simulink model "PV_Array_FLC"  (R2021a)
settings: Solver=VariableStepAuto  StartTime=0.0  StopTime=10.0  RelTol=1e-3
libraries: spsSeriesRLCBranchLib x3, spsDiodeLib x2, fuzblock x1, spsPWMGeneratorDCDCLib x1, spsMosfetLib x1, spsPVArrayLib x1, spsSeriesRLCLoadLib x1, spsVoltageMeasurementLib x1, spspowerguiLib x1
settings Model: Creator=admin  LastModifiedBy=admin

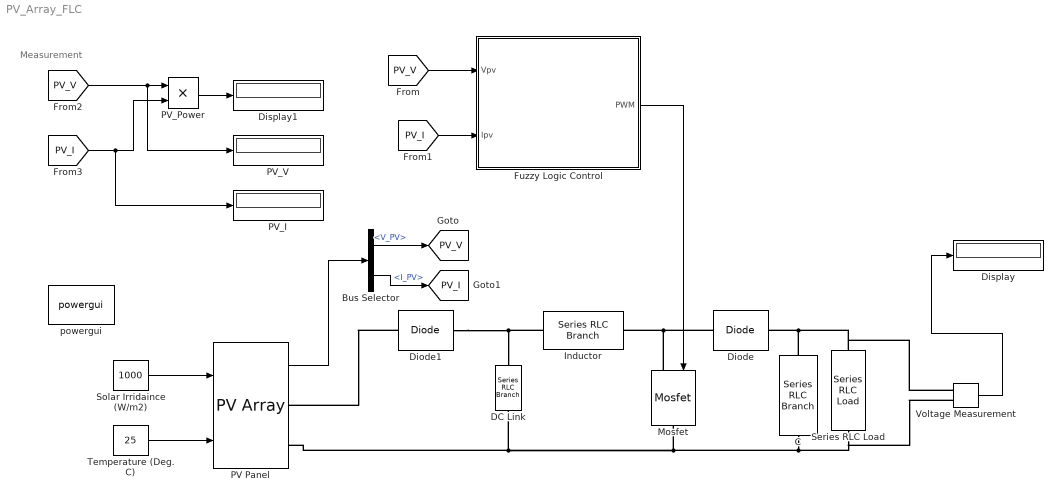
== system PV_Array_FLC ==
  note: Measurement
  Bus Selector : BusSelector  OutputSignals=V_PV,I_PV
  C : spsSeriesRLCBranchLib/Series RLC Branch  LConnTagsString=__new0  RConnTagsString=__new0  BranchType=C  Resistance=1  Inductance=1e-3  SetiL0=off  InitialCurrent=0  Capacitance=50e-6  Setx0=off  InitialVoltage=600  Measurements=None
  DC Link : spsSeriesRLCBranchLib/Series RLC Branch  LConnTagsString=__new0  RConnTagsString=__new0  BranchType=C  Resistance=0.001  Inductance=1.0  SetiL0=off  InitialCurrent=0  Capacitance=4000e-6  Setx0=off  InitialVoltage=310  Measurements=None
  Diode : spsDiodeLib/Diode  Ron=0.001  Lon=0  Vf=0.8  IC=0  UseSnubber=off  Rs=500  Cs=250e-9  Measurements=off
  Diode1 : spsDiodeLib/Diode  Ron=0.001  Lon=0  Vf=0.8  IC=0  UseSnubber=off  Rs=500  Cs=250e-9  Measurements=off
  Display : Display
  Display1 : Display
  "Fuzzy Logic Control " : Subsystem
  Inductor : spsSeriesRLCBranchLib/Series RLC Branch  LConnTagsString=__new0  RConnTagsString=__new0  BranchType=L  Resistance=0.01  Inductance=4e-4  SetiL0=off  InitialCurrent=5  Capacitance=1e-6  Setx0=off  InitialVoltage=0  Measurements=None
  Mosfet : spsMosfetLib/Mosfet  Ron=0.1  Lon=0  Rd=0.01  Vfd=0  IC=0  Rs=1e5  Cs=inf  Measurements=off
  "PV Panel  " : spsPVArrayLib/PV Array  Npar=1  Nser=2  PlotType=array @ 25 deg.C & specified irradiances  S_vec="[ 1000  500  100 ]"  Temp_C_vec="[ 45 25  ]"  ModuleName=Aavid Solar ASMS-220P  PlotWhenSelected=off  Pm=220.5  Ncell=60  Voc=36.8  Isc=8.08  Vm=30  Im=7.35  beta_Voc_pc=-0.3364  alpha_Isc_pc=0.038465  beta_Voc=-0.1238  alpha_Isc=0.003108  IL=8.1108  I0=1.1169e-10  nI=0.9567  Rsh=83.699  Rs=0.3192  RobustModel=off  RobustCellTemperature=313.3991  BAL=on  Tc=1e-6  Tfilter=5e-5
  PV_I : Display
  "PV_Power " : Product
  PV_V : Display
  Series RLC Load : spsSeriesRLCLoadLib/Series RLC Load  LConnTagsString=a  RConnTagsString=__new0  NominalVoltage=30  NominalFrequency=50  ActivePower=120  InductivePower=0  CapacitivePower=0  Setx0=off  InitialVoltage=0  SetiL0=off  InitialCurrent=0  Measurements=None  LoadType=constant Z
  Solar Irridaince (W/m2) : Constant  Value=1000
  Temperature (Deg. C) : Constant  Value=25
  Voltage Measurement : spsVoltageMeasurementLib/Voltage Measurement  PhasorSimulation=off  OutputType=Complex  PSBequivalent=0
  powergui : spspowerguiLib/powergui  Priority=1  SimulationMode=Discrete  SampleTime=5e-7  frequency=60  Iterations=50  frequencyindice=0  Pbase=100e6  ErrMax=1e-4  UnitsV=kV  UnitsW=MW  buscounter=0  FunctionMessages=off  echomessages=off  EnableUseOfTLC=off  CurrentSourceSwitches=off  DisableSnubberDevices=off  DisableRonSwitches=off  DisableVfSwitches=off  DisplayEquations=off  AutomaticDiscreteSolvers=off  SolverType=Tustin/Backward Euler (TBE)  Interpol=off  ExternalGateDelay=off  methode=off  Ts=100  x0status=blocks  SPID=off  SwTol=0  HookPort=off  NonlinearTolerance=1e-4  nMaxIteration=100  ContinueOnMaxIteration=off  RestoreLinks=warning  ResistiveCurrentMeasurement=off  Frange=[0:2:500]  Ylog=off  Xlog=on  ShowGrid=off  save=off  variable=ZData  structure=0  ZoomFFT=off  StartTime=0.0  cycles=1  DisplayStyle=1  fundamental=60  FreqAxis=off  MaxFrequency=1000  frequencyindicesteady=1  RmsSteady=1  display=off
  tag scope: PV_I=global, PV_V=global
  wires:
  "Fuzzy Logic Control "/1(PWM) -> Mosfet/1
  Temperature (Deg. C)/1 -> "PV Panel  "/2
  Solar Irridaince (W/m2)/1 -> "PV Panel  "/1
  Bus Selector/1 -> [PV_V]  "<V_PV>"
  Bus Selector/2 -> [PV_I]  "<I_PV>"
  [PV_V] -> "Fuzzy Logic Control "/1(Vpv)
  [PV_I] -> "Fuzzy Logic Control "/2(Ipv)
  "PV Panel  "/1 -> Bus Selector/1
  [PV_V] -> PV_V/1, "PV_Power "/1
  [PV_I] -> PV_I/1, "PV_Power "/2
  "PV_Power "/1 -> Display1/1
  Voltage Measurement/1 -> Display/1
  connections:
  Mosfet/RConn1 -- Voltage Measurement/LConn2 -- Series RLC Load/RConn1 -- C/RConn1 -- DC Link/RConn1 -- "PV Panel  "/RConn2
  C/LConn1 -- Voltage Measurement/LConn1 -- Series RLC Load/LConn1 -- Diode/RConn1
  Diode1/RConn1 -- DC Link/LConn1 -- Inductor/LConn1
  Mosfet/LConn1 -- Inductor/RConn1 -- Diode/LConn1
  Diode1/LConn1 -- "PV Panel  "/RConn1

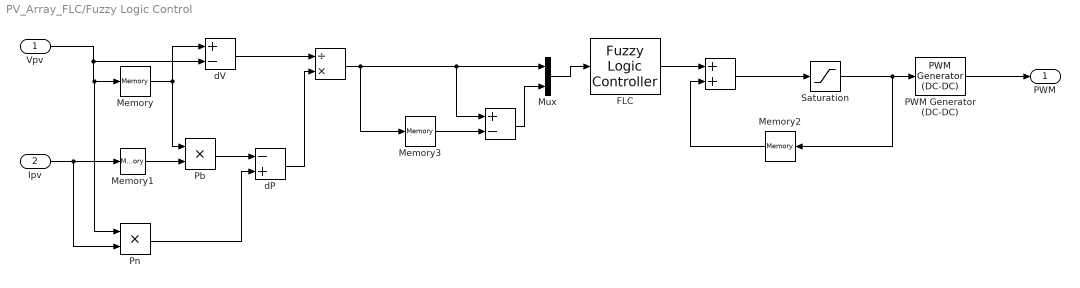
== system PV_Array_FLC/Fuzzy Logic Control  ==
  Vpv : Inport
  Ipv : Inport  Port=2
  "  " : Sum  Inputs=+-
  "   " : Sum
  "    " : Product  Inputs=/*
  "FLC " : fuzblock/Fuzzy Logic  Controller  FIS='tipper.fis'  OutputSampleNumber=101  DataType=double  FuzzifiedInputs=off  RuleFiringStrengths=off  RuleOutputs=off  AggregatedOutputs=off  SimulateUsing=Interpreted execution  OutOfRangeInputValueMessage=warning  NoRuleFiredMessage=warning  EmptyOutputFuzzySetMessage=warning
  "Memory " : Memory  InheritSampleTime=on
  "Memory1 " : Memory  InheritSampleTime=on
  Memory2 : Memory  InheritSampleTime=on
  Memory3 : Memory  InheritSampleTime=on
  Mux : Mux  Inputs=2
  PWM Generator (DC-DC) : spsPWMGeneratorDCDCLib/PWM Generator (DC-DC)  Fsw=15000  Ts=0
  Pb : Product
  Pn : Product
  Saturation : Saturate  UpperLimit=0.95  LowerLimit=0.1
  dP : Sum  Inputs=-+
  dV : Sum  Inputs=+-
  PWM : Outport
  wires:
  "Memory "/1 -> dV/1, Pb/1
  Ipv/1 -> Pn/2, "Memory1 "/1
  "Memory1 "/1 -> Pb/2
  Pb/1 -> dP/1
  Pn/1 -> dP/2
  Mux/1 -> "FLC "/1
  Memory2/1 -> "   "/2
  Memory3/1 -> "  "/2
  "  "/1 -> Mux/2
  PWM Generator (DC-DC)/1 -> PWM/1
  Vpv/1 -> dV/2, Pn/1, "Memory "/1
  dP/1 -> "    "/2
  "    "/1 -> Mux/1, "  "/1, Memory3/1
  dV/1 -> "    "/1
  Saturation/1 -> Memory2/1, PWM Generator (DC-DC)/1
  "FLC "/1 -> "   "/1
  "   "/1 -> Saturation/1
